simulink model "Dynamic_model_IM"  (R2013b)
settings: Solver=ode45  StartTime=0.0  StopTime=1  MaxStep=0.2e-3  RelTol=1e-6
values from neighbouring files (symbols this model uses):
  In = 5.1    [im_data.m]
  J = jm    (= 0.0069)    [im_data.m]
  Llr = 12.29e-3    (= 0.01229)    [im_data.m]
  Lls = 9.2e-3    (= 0.0092)    [im_data.m]
  Lm = 235.0e-3    (= 0.235)    [im_data.m]
  Omega_r = 2*pi*nn/60*p    (= 299.498499642)    [im_data.m]
  Omega_t = 0    [im_data.m]
  Omegae = 2*pi*fn    (= 314.159265359)    [im_data.m]
  p = 2.0    (= 2)    [im_data.m]
  Rr = 2.32    [im_data.m]
  Rs = 3.67*1.0    (= 3.67)    [im_data.m]
  Un = 220    [im_data.m]
libraries: simulink x1
Description:
  | Induction machine model as in Kaz. p 34
  | 
  | Note errors in (1.128) for rotor equations (Lm->Lr for some terms)!
settings Model: ExtModeTrigMode=oneshot  ExtModeArmWhenConnect=off  Creator=Michael M. Bech  LastModifiedBy=Fitim k
settings DataIOCC: LimitDataPoints=off  SignalLoggingSaveFormat=ModelDataLogs
settings OptimizationCC: BlockReduction=off  BooleanDataType=off  ExpressionDepthLimit=2147483647  InitFltsAndDblsToZero=on
settings DebuggingCC: SaveWithParameterizedLinksMsg=none  SignalResolutionControl=TryResolveAllWithWarning  SolverPrmCheckMsg=none  MultiTaskDSMMsg=warning  MultiTaskCondExecSysMsg=none  FcnCallInpInsideContextMsg=UseLocalSettings  StateNameClashWarn=warning
settings HardwareCC: TargetUnknown=on
settings RTWCC: IncludeERTFirstTime=on
settings GRTTargetCC: TargetFcnLib=ansi_tfl_tmw.mat  CombineOutputUpdateFcns=off  GRTInterface=on

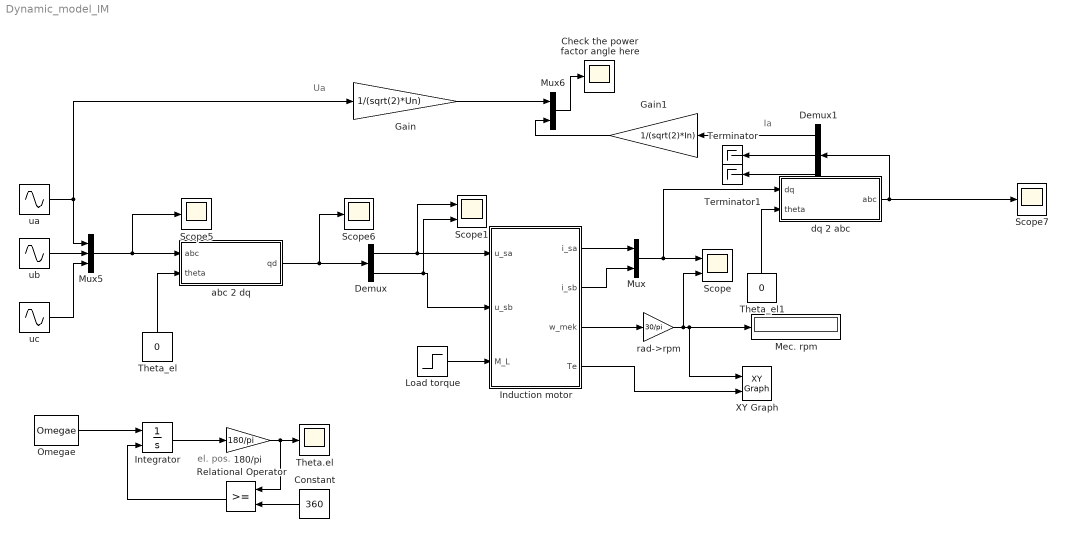
== system Dynamic_model_IM ==
  note: el. pos.
  note: Ua
  note: Ia
  180/pi : Gain  Gain=180/pi
  Check the power factor angle here : Scope
      settings: SaveName=ScopeData9
  Constant : Constant  Value=360
  Demux : Demux  Outputs=2
  Demux1 : Demux  Outputs=3
  Gain : Gain  Gain=1/(sqrt(2)*Un)
  Gain1 : Gain  Gain=1/(sqrt(2)*In)
  Induction motor : Subsystem
  Integrator : Integrator  ExternalReset=rising
  Load torque : Step  Time=0.25  After=14.6912  SampleTime=0
  Mec. rpm : Display
  Mux : Mux  Inputs=2
  Mux5 : Mux  Inputs=3
  Mux6 : Mux  Inputs=2
  Omegae : Constant  Value=Omegae
  Relational Operator : RelationalOperator  OutDataTypeStr=boolean
  Scope : Scope  NumInputPorts=2
      settings: TimeRange=0.5  YMin=-40~0  YMax=40~1750
  Scope1 : Scope  NumInputPorts=2
      settings: YMin=-50~-400  YMax=350~300  SaveName=ScopeData2
  Scope5 : Scope
      settings: SaveName=ScopeData5
  Scope6 : Scope
      settings: SaveName=ScopeData7
  Scope7 : Scope
      settings: SaveName=ScopeData8
  Terminator : Terminator
  Terminator1 : Terminator
  Theta.el : Scope
      settings: YMin=-225  YMax=225  SaveName=ScopeData6
  Theta_el : Constant  Value=0
  Theta_el1 : Constant  Value=0
  XY Graph : simulink/Sinks/XY Graph  xmin=0  xmax=2000  ymin=-5  ymax=50  st=-1
  abc 2 dq : Subsystem
  dq 2 abc : Subsystem
  rad->rpm : Gain  Gain=30/pi  SaturateOnIntegerOverflow=on  OutDataTypeStr=Inherit: Same as input  ParamDataTypeStr=Inherit: Same as input
  ua : Sin  Amplitude=sqrt(2)*Un  Frequency=Omegae  Phase=pi/2  SampleTime=0
  ub : Sin  Amplitude=sqrt(2)*Un  Frequency=Omegae  Phase=pi/2-120/180*pi  SampleTime=0
  uc : Sin  Amplitude=sqrt(2)*Un  Frequency=Omegae  Phase=pi/2-240/180*pi  SampleTime=0
  wires:
  Induction motor/1(i_sa) -> Mux/1
  Induction motor/2(i_sb) -> Mux/2
  Mux/1 -> Scope/1, dq 2 abc/1(dq)
  Induction motor/3(w_mek) -> rad->rpm/1
  rad->rpm/1 -> XY Graph/1, Mec. rpm/1, Scope/2
  abc 2 dq/1(qd) -> Demux/1, Scope6/1
  Demux/2 -> Scope1/2, Induction motor/2(u_sb)
  ua/1 -> Mux5/1, Gain/1
  uc/1 -> Mux5/3
  ub/1 -> Mux5/2
  Mux5/1 -> abc 2 dq/1(abc), Scope5/1
  Integrator/1 -> 180/pi/1
  180/pi/1 -> Theta.el/1, Relational Operator/1
  Constant/1 -> Relational Operator/2
  Relational Operator/1 -> Integrator/2
  Omegae/1 -> Integrator/1
  Theta_el/1 -> abc 2 dq/2(theta)
  Demux/1 -> Scope1/1, Induction motor/1(u_sa)
  Theta_el1/1 -> dq 2 abc/2(theta)
  dq 2 abc/1(abc) -> Scope7/1, Demux1/1
  Mux6/1 -> Check the power factor angle here/1
  Gain/1 -> Mux6/1
  Demux1/2 -> Terminator/1
  Demux1/3 -> Terminator1/1
  Demux1/1 -> Gain1/1
  Gain1/1 -> Mux6/2
  Induction motor/4(Te) -> XY Graph/2
  Load torque/1 -> Induction motor/3(M_L)

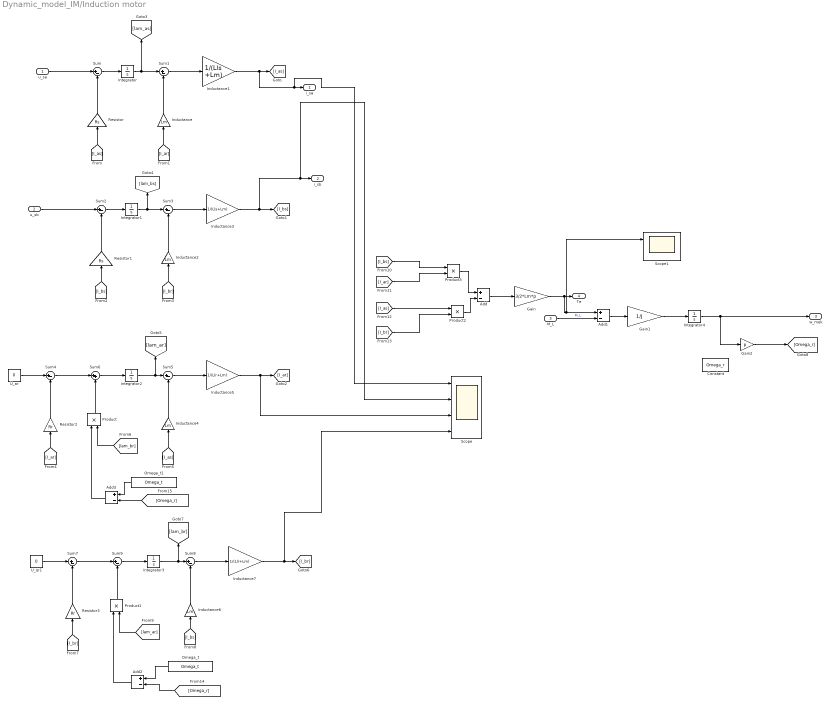
== system Dynamic_model_IM/Induction motor ==
  u_sa : Inport
  u_sb : Inport  Port=2
  M_L : Inport  Port=3
  Add{,1..3} (4 alike) : Sum  Inputs=+-
  Constant : Constant  Value=Omega_r
  Gain : Gain  Gain=3/2*Lm*p
  Gain1 : Gain  Gain=1/J
  Gain2 : Gain  Gain=p
  Inductance{,2,4,6} (4 alike) : Gain  Gain=Lm
  Inductance1 : Gain  Gain=1/(Lls +Lm)
  Inductance3 : Gain  Gain=1/(Lls+Lm)
  Inductance5 : Gain  Gain=1/(Llr+Lm)
  Inductance7 : Gain  Gain=1/(Llr+Lm)
  Integrator{,1..4} (5 alike) : Integrator
  Omega_t : Constant  Value=Omega_t
  Omega_t1 : Constant  Value=Omega_t
  Product{,1..3} (4 alike) : Product
  Resistor : Gain  Gain=Rs
  Resistor1 : Gain  Gain=Rs
  Resistor2 : Gain  Gain=Rr
  Resistor3 : Gain  Gain=Rr
  Scope : Scope  NumInputPorts=4
      settings: YMin=-3.5e+14~-3.5e+14~0~0  YMax=0~0~3.75e+14~3.75e+14
  Scope1 : Scope  NumInputPorts=2
      settings: YMin=-3.5e+14~-3.5e+14  YMax=0~0  SaveName=ScopeData3
  Sum{,1..5,7..9} (9 alike) : Sum  Inputs=|+-
  Sum6 : Sum  Inputs=|++
  U_ar : Constant  Value=0
  U_qr1 : Constant  Value=0
  i_sa : Outport
  i_sb : Outport  Port=2
  w_mek : Outport  Port=3
  Te : Outport  Port=4
  wires:
  Resistor/1 -> Sum/2
  Sum/1 -> Integrator/1
  Integrator/1 -> Sum1/1, [lam_as]
  Inductance/1 -> Sum1/2
  Sum1/1 -> Inductance1/1
  Inductance1/1 -> Scope/1, i_sa/1, [I_as]
  [I_as] -> Resistor/1
  [I_ar] -> Inductance/1
  Resistor1/1 -> Sum2/2
  Sum2/1 -> Integrator1/1
  Integrator1/1 -> Sum3/1, [lam_bs]
  Inductance2/1 -> Sum3/2
  Sum3/1 -> Inductance3/1
  Inductance3/1 -> Scope/2, i_sb/1, [I_bs]
  [I_bs] -> Resistor1/1
  [I_br] -> Inductance2/1
  U_ar/1 -> Sum4/1
  Resistor2/1 -> Sum4/2
  Integrator2/1 -> Sum5/1, [lam_ar]
  Inductance4/1 -> Sum5/2
  Sum5/1 -> Inductance5/1
  Inductance5/1 -> Scope/3, [I_ar]
  [I_ar] -> Resistor2/1
  [I_as] -> Inductance4/1
  Sum4/1 -> Sum6/1
  Sum6/1 -> Integrator2/1
  Product/1 -> Sum6/2
  [lam_br] -> Product/2
  Add3/1 -> Product/1
  U_qr1/1 -> Sum7/1
  Resistor3/1 -> Sum7/2
  Integrator3/1 -> Sum8/1, [lam_br]
  Inductance6/1 -> Sum8/2
  Sum8/1 -> Inductance7/1
  Inductance7/1 -> Scope/4, [I_br]
  [I_br] -> Resistor3/1
  [I_bs] -> Inductance6/1
  Sum7/1 -> Sum9/1
  Sum9/1 -> Integrator3/1
  Product1/1 -> Sum9/2
  [lam_ar] -> Product1/2
  Add2/1 -> Product1/1
  u_sb/1 -> Sum2/1
  u_sa/1 -> Sum/1
  Add/1 -> Gain/1
  [I_bs] -> Product3/1
  [I_ar] -> Product3/2
  [I_as] -> Product2/1
  [I_br] -> Product2/2
  Product2/1 -> Add/2
  Product3/1 -> Add/1
  Gain/1 -> Add1/1, Scope1/1, Te/1
  Add1/1 -> Gain1/1
  Gain1/1 -> Integrator4/1
  Integrator4/1 -> w_mek/1, Gain2/1
  [Omega_r] -> Add2/2
  Omega_t/1 -> Add2/1
  [Omega_r] -> Add3/2
  Omega_t1/1 -> Add3/1
  M_L/1 -> Add1/2  "M_L"
  Gain2/1 -> [Omega_r]

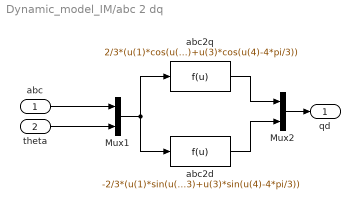
== system Dynamic_model_IM/abc 2 dq ==
  abc : Inport
  theta : Inport  Port=2
  Mux1 : Mux  Inputs=2
  Mux2 : Mux  Inputs=2
  abc2d : Fcn  Expr=-2/3*(u(1)*sin(u(4))+u(2)*sin(u(4)-2*pi/3)+u(3)*sin(u(4)-4*pi/3))
  abc2q : Fcn  Expr=2/3*(u(1)*cos(u(4))+u(2)*cos(u(4)-2*pi/3)+u(3)*cos(u(4)-4*pi/3))
  qd : Outport
  wires:
  abc/1 -> Mux1/1
  theta/1 -> Mux1/2
  Mux1/1 -> abc2q/1, abc2d/1
  abc2q/1 -> Mux2/1
  abc2d/1 -> Mux2/2
  Mux2/1 -> qd/1

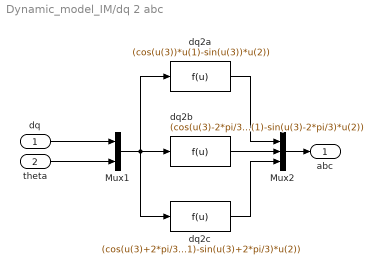
== system Dynamic_model_IM/dq 2 abc ==
  dq : Inport
  theta : Inport  Port=2
  Mux1 : Mux  Inputs=2
  Mux2 : Mux  Inputs=3
  dq2a : Fcn  Expr=(cos(u(3))*u(1)-sin(u(3))*u(2))
  dq2b : Fcn  Expr=(cos(u(3)-2*pi/3)*u(1)-sin(u(3)-2*pi/3)*u(2))
  dq2c : Fcn  Expr=(cos(u(3)+2*pi/3)*u(1)-sin(u(3)+2*pi/3)*u(2))
  abc : Outport
  wires:
  Mux2/1 -> abc/1
  dq2b/1 -> Mux2/2
  dq2a/1 -> Mux2/1
  Mux1/1 -> dq2a/1, dq2c/1, dq2b/1
  theta/1 -> Mux1/2
  dq/1 -> Mux1/1
  dq2c/1 -> Mux2/3
